simulink model "Wind_DC_Battery_Complete"  (R2022a)
settings: Solver=daessc  StartTime=0.0  StopTime=3600*24  MaxStep=60/10  RelTol=1e-3  AbsTol=1e-3
undefined symbols (not defined in the file or in its folder): Battery, Electric, Generator, Plate, R_h2, Setpoint
libraries: fl_lib x63, nesl_utility x18, ee_lib x5, simulink x1, sdl_lib x1
(part 5 of 5)

== matlab function Wind_DC_Battery_Complete/Electrolyzer/Sensor/MATLAB Function ==
  data: u input; Z output
function Z = fcn(u)

Z = min(u(2)/u(1),1e3);
